simulink model "gyroscope"  (R2015a)
settings: Solver=ode45  StartTime=0.0  StopTime=10  RelTol=1e-3
model workspace (MAT data in the model file):
  randomSeed = 0
undefined symbols (not defined in the file): gyroMax, gyroOffset
libraries: simulink x1, dsparch4 x1
settings Model: ParameterArgumentNames=randomSeed  Creator=johnz  LastModifiedBy=johnz

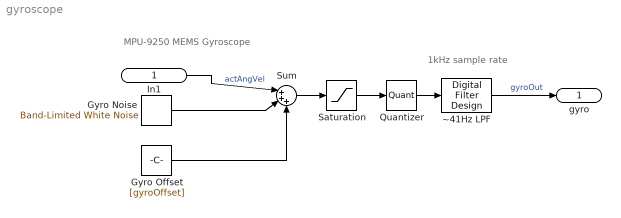
== system gyroscope ==
  note: MPU-9250 MEMS Gyroscope
  note: 1kHz sample rate
  In1 : Inport
  Gyro Noise : simulink/Sources/Band-Limited White Noise  Cov=gyroNoise  Ts=1/1000  seed=randomSeed
  Gyro Offset : Constant  Value=[gyroOffset]
  Quantizer : Quantizer  QuantizationInterval=gyroSensitivity
  Saturation : Saturate  UpperLimit=gyroMax  LowerLimit=-gyroMax
  Sum : Sum  Inputs=|+++
  "~41Hz LPF " : dsparch4/Digital Filter Design  mwdsp_browser_bugfix_var=off
  gyro : Outport  OutDataTypeStr=double  PortDimensions=1
  wires:
  In1/1 -> Sum/1  "actAngVel"
  Sum/1 -> Saturation/1
  Saturation/1 -> Quantizer/1
  Quantizer/1 -> "~41Hz LPF "/1
  Gyro Offset/1 -> Sum/3
  Gyro Noise/1 -> Sum/2
  "~41Hz LPF "/1 -> gyro/1  "gyroOut"
